simulink model "assignment1"  (R2020a)
settings: Solver=FixedStepDiscrete  StartTime=0.0  StopTime=10.0  FixedStep=0.001  RelTol=1e-3  EnableMultiTasking=on
undefined symbols (not defined in the file): D0, D1, D10, D11, D12, D13, D2, D3, D4, D5, D6, D7, D8, D9, PTA0, PTA1, PTA2, PTB23, PTB9, PTC16, PTC17, PTC2, PTC3, PTC4, PTD0, PTD1, PTD2, PTD3
libraries: frdmk64flib x18
settings Model: ExtModeTrigDuration=5  Creator=Nick  LastModifiedBy=Nick
settings OptimizationCC: EnhancedBackFolding=on  PassReuseOutputArgsAs=Individual arguments  ZeroExternalMemoryAtStartup=off  ZeroInternalMemoryAtStartup=off  MaxStackSize=64  OptimizeBlockOrder=speed  DifferentSizesBufferReuse=on  OptimizationCustomize=off  EfficientTunableParamExpr=on
settings DebuggingCC: ParameterTunabilityLossMsg=error
settings HardwareCC: ProdBitPerPointer=32  ProdBitPerSizeT=32  ProdBitPerPtrDiffT=32  ProdLargestAtomicInteger=Long  ProdLargestAtomicFloat=Double  ProdWordSize=32  ProdHWDeviceType=ARM Compatible->ARM Cortex
settings SFSimCC: MATLABDynamicMemAlloc=off
settings RTWCC: SystemTargetFile=ert.tlc  HardwareBoard=NXP FRDM-K64F  TemplateMakefile=ert_default_tmf  Toolchain=GNU Tools for ARM Embedded Processors
settings CodeAppCC: ForceParamTrailComments=on  IgnoreCustomStorageClasses=off  OperatorAnnotations=on  SimulinkDataObjDesc=on  SFDataObjDesc=on  InsertBlockDesc=on

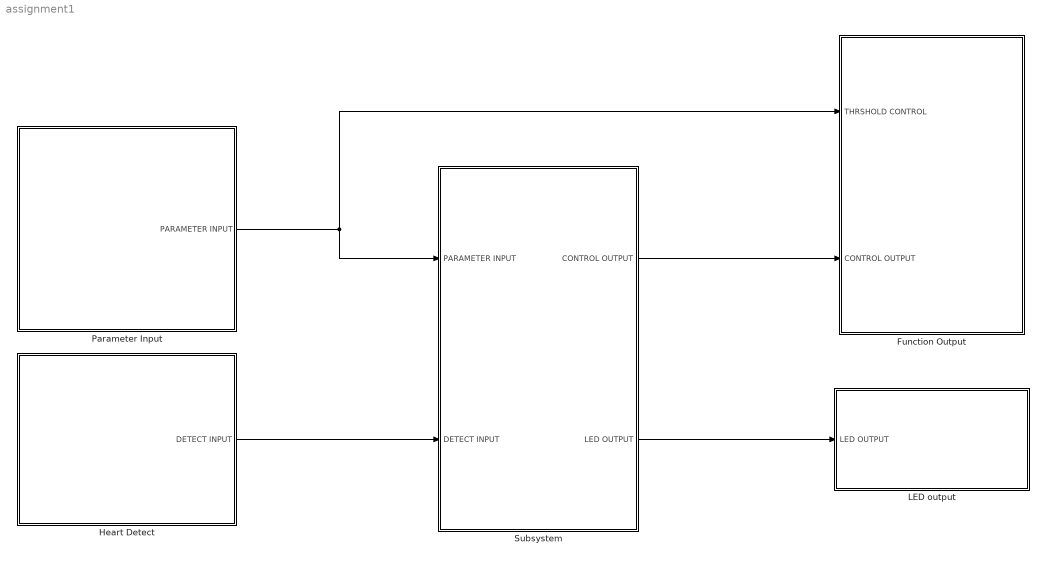
== system assignment1 ==
  Function Output : Subsystem
  Heart Detect : Subsystem
  LED output : Subsystem
  Parameter Input : Subsystem
  Subsystem : Subsystem
  wires:
  Parameter Input/1(PARAMETER INPUT) -> Function Output/1(THRSHOLD CONTROL), Subsystem/1(PARAMETER INPUT)
  Heart Detect/1(DETECT INPUT) -> Subsystem/2(DETECT INPUT)
  Subsystem/1(CONTROL OUTPUT) -> Function Output/2(CONTROL OUTPUT)
  Subsystem/2(LED OUTPUT) -> LED output/1(LED OUTPUT)

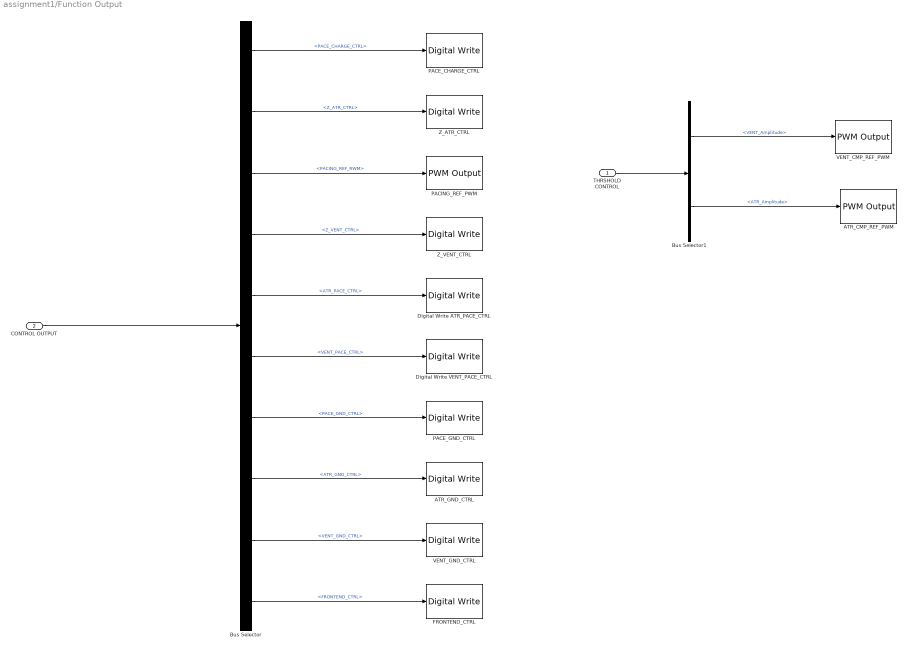
== system assignment1/Function Output ==
  THRSHOLD CONTROL : Inport
  CONTROL OUTPUT : Inport  Port=2
  ATR_CMP_REF_PWM : frdmk64flib/PWM Output  Whichpin=PTC2 (D6)  InitialFrequency=2000  InitialDutyCycle=0
  ATR_GND_CTRL : frdmk64flib/Digital Write  Whichpin=PTD2 (D11)
  Bus Selector : BusSelector  OutputSignals=PACE_CHARGE_CTRL,Z_ATR_CTRL,PACING_REF_RWM,Z_VENT_CTRL,ATR_PACE_CTRL,VENT_PACE_CTRL,PACE_GND_CTRL,ATR_GND_CTRL,VENT_GND_CTRL,FRONTEND_CTRL
  Bus Selector1 : BusSelector  OutputSignals=VENT_Amplitude,ATR_Amplitude
  Digital Write ATR_PACE_CTRL : frdmk64flib/Digital Write  Whichpin=PTA0 (D8)
  Digital Write VENT_PACE_CTRL : frdmk64flib/Digital Write  Whichpin=PTC4 (D9)
  FRONTEND_CTRL : frdmk64flib/Digital Write  Whichpin=PTD1 (D13)
  PACE_CHARGE_CTRL : frdmk64flib/Digital Write  Whichpin=PTB9 (D2)
  PACE_GND_CTRL : frdmk64flib/Digital Write  Whichpin=PTD0 (D10)
  PACING_REF_PWM : frdmk64flib/PWM Output  Whichpin=PTA2 (D5)  InitialFrequency=2000  InitialDutyCycle=0
  VENT_CMP_REF_PWM : frdmk64flib/PWM Output  Whichpin=PTA1 (D3)  InitialFrequency=2000  InitialDutyCycle=0
  VENT_GND_CTRL : frdmk64flib/Digital Write  Whichpin=PTD3 (D12)
  Z_ATR_CTRL : frdmk64flib/Digital Write  Whichpin=PTB23 (D4)
  Z_VENT_CTRL : frdmk64flib/Digital Write  Whichpin=PTC3 (D7)
  wires:
  CONTROL OUTPUT/1 -> Bus Selector/1
  Bus Selector/1 -> PACE_CHARGE_CTRL/1  "<PACE_CHARGE_CTRL>"
  Bus Selector/2 -> Z_ATR_CTRL/1  "<Z_ATR_CTRL>"
  Bus Selector/3 -> PACING_REF_PWM/1  "<PACING_REF_RWM>"
  Bus Selector/4 -> Z_VENT_CTRL/1  "<Z_VENT_CTRL>"
  Bus Selector/5 -> Digital Write ATR_PACE_CTRL/1  "<ATR_PACE_CTRL>"
  Bus Selector/6 -> Digital Write VENT_PACE_CTRL/1  "<VENT_PACE_CTRL>"
  Bus Selector/7 -> PACE_GND_CTRL/1  "<PACE_GND_CTRL>"
  Bus Selector/8 -> ATR_GND_CTRL/1  "<ATR_GND_CTRL>"
  Bus Selector/9 -> VENT_GND_CTRL/1  "<VENT_GND_CTRL>"
  Bus Selector/10 -> FRONTEND_CTRL/1  "<FRONTEND_CTRL>"
  THRSHOLD CONTROL/1 -> Bus Selector1/1
  Bus Selector1/1 -> VENT_CMP_REF_PWM/1  "<VENT_Amplitude>"
  Bus Selector1/2 -> ATR_CMP_REF_PWM/1  "<ATR_Amplitude>"

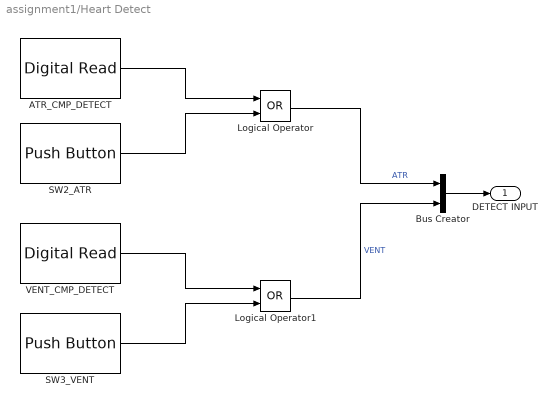
== system assignment1/Heart Detect ==
  ATR_CMP_DETECT : frdmk64flib/Digital Read  Whichpin=PTC16 (D0)  SampleTime=-1
  Bus Creator : BusCreator  Inputs=2
  Logical Operator : Logic  Operator=OR  AllPortsSameDT=off  OutDataTypeStr=boolean
  Logical Operator1 : Logic  Operator=OR  AllPortsSameDT=off  OutDataTypeStr=boolean
  SW2_ATR : frdmk64flib/Push Button  Whichswitch=SW2  SampleTime1=-1
  SW3_VENT : frdmk64flib/Push Button  Whichswitch=SW3  SampleTime1=-1
  VENT_CMP_DETECT : frdmk64flib/Digital Read  Whichpin=PTC17 (D1)  SampleTime=-1
  DETECT INPUT : Outport
  wires:
  ATR_CMP_DETECT/1 -> Logical Operator/1
  SW2_ATR/1 -> Logical Operator/2
  SW3_VENT/1 -> Logical Operator1/2
  VENT_CMP_DETECT/1 -> Logical Operator1/1
  Logical Operator/1 -> Bus Creator/1  "ATR"
  Logical Operator1/1 -> Bus Creator/2  "VENT"
  Bus Creator/1 -> DETECT INPUT/1

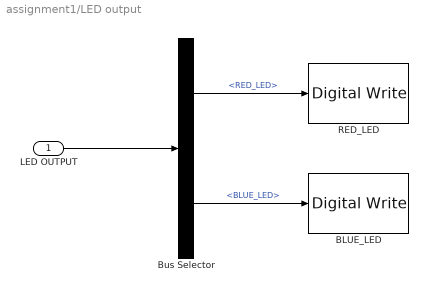
== system assignment1/LED output ==
  LED OUTPUT : Inport
  BLUE_LED : frdmk64flib/Digital Write  Whichpin=BLUE_LED
  Bus Selector : BusSelector  OutputSignals=RED_LED,BLUE_LED
  RED_LED : frdmk64flib/Digital Write  Whichpin=RED_LED
  wires:
  Bus Selector/1 -> RED_LED/1  "<RED_LED>"
  Bus Selector/2 -> BLUE_LED/1  "<BLUE_LED>"
  LED OUTPUT/1 -> Bus Selector/1

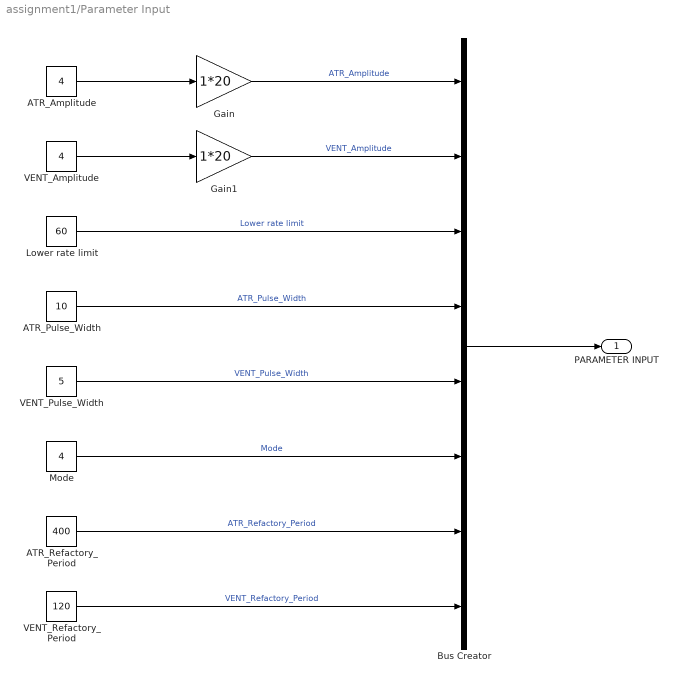
== system assignment1/Parameter Input ==
  ATR_Amplitude : Constant  Value=4
  ATR_Pulse_Width : Constant  Value=10
  ATR_Refactory_Period : Constant  Value=400
  Bus Creator : BusCreator  Inputs=8
  Gain : Gain  Gain=1*20
  Gain1 : Gain  Gain=1*20
  Lower rate limit : Constant  Value=60
  Mode : Constant  Value=4
  VENT_Amplitude : Constant  Value=4
  VENT_Pulse_Width : Constant  Value=5
  VENT_Refactory_Period : Constant  Value=120
  PARAMETER INPUT : Outport
  wires:
  ATR_Amplitude/1 -> Gain/1
  VENT_Amplitude/1 -> Gain1/1
  Gain/1 -> Bus Creator/1  "ATR_Amplitude"
  Gain1/1 -> Bus Creator/2  "VENT_Amplitude"
  Lower rate limit/1 -> Bus Creator/3  "Lower rate limit"
  ATR_Pulse_Width/1 -> Bus Creator/4  "ATR_Pulse_Width"
  VENT_Pulse_Width/1 -> Bus Creator/5  "VENT_Pulse_Width"
  Mode/1 -> Bus Creator/6  "Mode"
  ATR_Refactory_Period/1 -> Bus Creator/7  "ATR_Refactory_Period"
  VENT_Refactory_Period/1 -> Bus Creator/8  "VENT_Refactory_Period"
  Bus Creator/1 -> PARAMETER INPUT/1

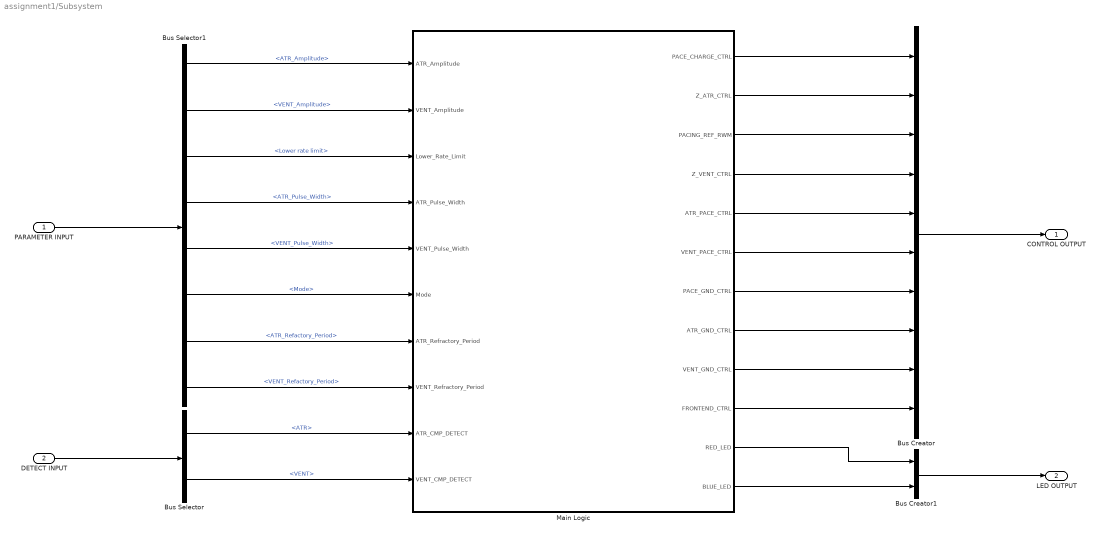
== system assignment1/Subsystem ==
  PARAMETER INPUT : Inport
  DETECT INPUT : Inport  Port=2
  Bus Creator : BusCreator  Inputs=10
  Bus Creator1 : BusCreator  Inputs=2
  Bus Selector : BusSelector  OutputSignals=ATR,VENT
  Bus Selector1 : BusSelector  OutputSignals=ATR_Amplitude,VENT_Amplitude,Lower rate limit,ATR_Pulse_Width,VENT_Pulse_Width,Mode,ATR_Refactory_Period,VENT_Refactory_Period
  Main Logic : Stateflow chart  TreatAsAtomicUnit=on  VariantControl=Choice
  CONTROL OUTPUT : Outport
  LED OUTPUT : Outport  Port=2
  wires:
  PARAMETER INPUT/1 -> Bus Selector1/1
  Bus Selector1/1 -> Main Logic/1(ATR_Amplitude)  "<ATR_Amplitude>"
  Bus Selector1/2 -> Main Logic/2(VENT_Amplitude)  "<VENT_Amplitude>"
  Bus Selector1/3 -> Main Logic/3(Lower_Rate_Limit)  "<Lower rate limit>"
  Bus Selector1/4 -> Main Logic/4(ATR_Pulse_Width)  "<ATR_Pulse_Width>"
  Bus Selector1/5 -> Main Logic/5(VENT_Pulse_Width)  "<VENT_Pulse_Width>"
  Bus Selector1/6 -> Main Logic/6(Mode)  "<Mode>"
  Bus Selector1/7 -> Main Logic/7(ATR_Refractory_Period)  "<ATR_Refactory_Period>"
  Bus Selector1/8 -> Main Logic/8(VENT_Refractory_Period)  "<VENT_Refactory_Period>"
  Bus Selector/1 -> Main Logic/9(ATR_CMP_DETECT)  "<ATR>"
  Bus Selector/2 -> Main Logic/10(VENT_CMP_DETECT)  "<VENT>"
  DETECT INPUT/1 -> Bus Selector/1
  Main Logic/1(PACE_CHARGE_CTRL) -> Bus Creator/1
  Main Logic/2(Z_ATR_CTRL) -> Bus Creator/2
  Main Logic/3(PACING_REF_RWM) -> Bus Creator/3
  Main Logic/4(Z_VENT_CTRL) -> Bus Creator/4
  Main Logic/5(ATR_PACE_CTRL) -> Bus Creator/5
  Main Logic/6(VENT_PACE_CTRL) -> Bus Creator/6
  Main Logic/7(PACE_GND_CTRL) -> Bus Creator/7
  Main Logic/8(ATR_GND_CTRL) -> Bus Creator/8
  Main Logic/9(VENT_GND_CTRL) -> Bus Creator/9
  Main Logic/10(FRONTEND_CTRL) -> Bus Creator/10
  Bus Creator/1 -> CONTROL OUTPUT/1
  Main Logic/11(RED_LED) -> Bus Creator1/1
  Main Logic/12(BLUE_LED) -> Bus Creator1/2
  Bus Creator1/1 -> LED OUTPUT/1

== stateflow chart assignment1/Subsystem/Main Logic ==
  state AV_Pacing_AOO
    entry:
    %
    PACE_CHARGE_CTRL = 0;
    %
    PACE_GND_CTRL = 1;
    ATR_PACE_CTRL = 1;
    ATR_GND_CTRL = 0;
    Z_ATR_CTRL = 0;
    Z_VENT_CTRL =0;
    %
    VENT_PACE_CTRL = 0;
    VENT_GND_CTRL = 0;
    %
    PACING_REF_RWM = ATR_Amplitude;
    RED_LED=1;
  state AOO
    %CHARGING_C22
    entry:
    ATR_PACE_CTRL = 0;
    VENT_PACE_CTRL = 0;
    %
    PACING_REF_RWM = ATR_Amplitude;
    PACE_CHARGE_CTRL = 1;
    %
    PACE_GND_CTRL = 1;
    Z_ATR_CTRL = 0;
    Z_VENT_CTRL = 0;
    %
    ATR_GND_CTRL = 1;
    VENT_GND_CTRL = 0;
    RED_LED=0;
  state AV_Pacing_VOO
    entry:
    %
    PACE_CHARGE_CTRL = 0;
    %
    PACE_GND_CTRL = 1;
    ATR_GND_CTRL = 0;
    ATR_PACE_CTRL = 0;
    Z_ATR_CTRL = 0;
    Z_VENT_CTRL =0;
    %
    VENT_PACE_CTRL = 1;
    VENT_GND_CTRL = 0;
    %
    PACING_REF_RWM = VENT_Amplitude;
    BLUE_LED=1;
  state VOO
    %CHARGING_C23
    entry:
    ATR_PACE_CTRL = 0;
    VENT_PACE_CTRL = 0;
    %
    PACING_REF_RWM = VENT_Amplitude;
    PACE_CHARGE_CTRL = 1;
    %
    PACE_GND_CTRL = 1;
    Z_ATR_CTRL = 0;
    Z_VENT_CTRL = 0;
    %
    ATR_GND_CTRL = 0;
    VENT_GND_CTRL = 1;
    %
    BLUE_LED=0;
  state MAIN
    entry:
    %disconnect the pacemaker
    PACE_CHARGE_CTRL = 0;
    VENT_PACE_CTRL = 0;
    ATR_PACE_CTRL = 0;
    PACE_GND_CTRL=0;
    ATR_GND_CTRL=0;
    VENT_GND_CTRL=0;
    Z_ATR_CTRL = 0;
    Z_VENT_CTRL = 0;
    %stop sensing
    FRONTEND_CTRL=0;
  state AAI
    %CHARGING_C22
    entry:
    ATR_PACE_CTRL = 0;
    VENT_PACE_CTRL = 0;
    %
    PACING_REF_RWM = ATR_Amplitude;
    PACE_CHARGE_CTRL = 1;
    %
    PACE_GND_CTRL = 1;
    Z_ATR_CTRL = 0;
    Z_VENT_CTRL = 0;
    %
    ATR_GND_CTRL = 1;
    VENT_GND_CTRL = 0;
    RED_LED=0;
    %star sensing
    FRONTEND_CTRL=1;
  state AV_Pacing_AAI
    entry:
    %stop sensing
    FRONTEND_CTRL=0;
    %
    PACE_CHARGE_CTRL = 0;
    %
    PACE_GND_CTRL = 1;
    ATR_PACE_CTRL = 1;
    ATR_GND_CTRL = 0;
    Z_ATR_CTRL = 0;
    Z_VENT_CTRL =0;
    %
    VENT_PACE_CTRL = 0;
    VENT_GND_CTRL = 0;
    %
    PACING_REF_RWM = ATR_Amplitude;
    RED_LED=1;
  state Refractory_ATR
    entry:
    FRONTEND_CTRL=0; %sensing off
  state AV_Pacing_VVI
    entry:
    %stop sensing
    FRONTEND_CTRL=0;
    %
    PACE_CHARGE_CTRL = 0;
    %
    PACE_GND_CTRL = 1;
    ATR_GND_CTRL = 0;
    ATR_PACE_CTRL = 0;
    Z_ATR_CTRL = 0;
    Z_VENT_CTRL =0;
    %
    VENT_PACE_CTRL = 1;
    VENT_GND_CTRL = 0;
    %
    PACING_REF_RWM = VENT_Amplitude;
    BLUE_LED=1;
  state VVI
    %CHARGING_C23
    ATR_PACE_CTRL = 0;
    VENT_PACE_CTRL = 0;
    %
    PACING_REF_RWM = VENT_Amplitude;
    PACE_CHARGE_CTRL = 1;
    %
    PACE_GND_CTRL = 1;
    Z_ATR_CTRL = 0;
    Z_VENT_CTRL = 0;
    %
    ATR_GND_CTRL = 0;
    VENT_GND_CTRL = 1;
    %
    BLUE_LED=0;
    %stop sensing
    FRONTEND_CTRL=1;
  state Refractory_VENT
    entry:
    FRONTEND_CTRL=0; %sensing off
  AOO -> AV_Pacing_AOO : after(60/Lower_Rate_Limit*1000 - ATR_Pulse_Width,msec)
  MAIN -> AOO [order 2] : [Mode == 1]
  AV_Pacing_AOO -> AOO : after(ATR_Pulse_Width,msec)
  AV_Pacing_VOO -> VOO : after(VENT_Pulse_Width,msec)
  MAIN -> VOO [order 1] : [Mode == 2]
  (default) -> MAIN
  VOO -> AV_Pacing_VOO : after((60/Lower_Rate_Limit)*1000 - VENT_Pulse_Width,msec)
  MAIN -> AAI [order 3] : [Mode == 3]
  MAIN -> VVI [order 4] : [Mode ==4 ]
  AAI -> AV_Pacing_AAI [order 1] : after(60/Lower_Rate_Limit * 1000 - ATR_Refractory_Period - ATR_Pulse_Width,msec)
  AAI -> (junction 70) [order 2] : [ATR_CMP_DETECT==true]
  (junction 70) -> Refractory_ATR
  AV_Pacing_AAI -> Refractory_ATR : after(ATR_Pulse_Width,msec)
  Refractory_ATR -> AAI : after(ATR_Refractory_Period,msec)
  VVI -> AV_Pacing_VVI [order 1] : after(60/Lower_Rate_Limit*1000 - VENT_Refractory_Period - VENT_Pulse_Width,msec)
  VVI -> (junction 85) [order 2] : [VENT_CMP_DETECT==true]
  (junction 85) -> Refractory_VENT
  Refractory_VENT -> VVI : after(VENT_Refractory_Period,msec)
  AV_Pacing_VVI -> Refractory_VENT : after(VENT_Pulse_Width,msec)
  data: PACE_CHARGE_CTRL output; Z_ATR_CTRL output; PACING_REF_RWM output; Z_VENT_CTRL output; ATR_PACE_CTRL output; VENT_PACE_CTRL output; PACE_GND_CTRL output; ATR_GND_CTRL output; VENT_GND_CTRL output; FRONTEND_CTRL output; RED_LED output; ATR_Amplitude input; VENT_Amplitude input; Lower_Rate_Limit input; ATR_Pulse_Width input; VENT_Pulse_Width input; Mode input; ATR_Refractory_Period input; VENT_Refractory_Period input; BLUE_LED output; ATR_CMP_DETECT input; VENT_CMP_DETECT input
